simulink model "saturn_ib_stack_test"  (Simulink 6.2)
settings: Solver=ode4  SolverMode=SingleTasking  StartTime=-20.0  StopTime=620  FixedStep=0.005  RelTol=1e-3
values from neighbouring files (symbols this model uses):
  A_z_deg = 82.8200    (= 82.82)    [AS205_presettings.m]
  BN_1_sec = 14.4    [AS205_presettings.m]
  DeltaV_b_mps = 7.2381    [AS205_presettings.m]
  epsilon_2_sec = 15.0    (= 15)    [AS205_presettings.m]
  epsilon_prime_sec = 3.0    (= 3)    [AS205_presettings.m]
  i_deg = 28.89597    [AS205_presettings.m]
  lambda_0_deg = 102.32900    (= 102.329)    [AS205_presettings.m]
  lambda_L_deg = -80.561141    [AS205_presettings.m]
  pad_roll_L_deg = 100.0    (= 100)    [AS205_presettings.m]
  phi_L_deg = 28.521963    [AS205_presettings.m]
  phi_L_prime_deg = 28.360795    [AS205_presettings.m]
  R_L_m = 6373385.0    (= 6373385)    [AS205_presettings.m]
  R_T_m = 6570774.0    (= 6570774)    [AS205_presettings.m]
  T3_FM_sec = 6.08    [AS205_presettings.m]
  T_HSL_sec = 5.0    (= 5)    [AS205_presettings.m]
  Theta_T_deg = 0.000    (= 0)    [AS205_presettings.m]
  V_T_mps = 7780.976    [AS205_presettings.m]
  Xdotdot_VGT_mps2 = -9.251    [AS205_presettings.m]
undefined symbols (not defined in the file or in its folder): e0_0, e1_0, e2_0, e3_0, m, s
libraries: simulink x99, aerolibconvert x83, aerolibutil x63, aerolibtransform2 x34, aerolibasang x2, aerolibatmos2 x2, aerolib6dofsys x2
(part 2 of 7)

== system saturn_ib_stack_test/Saturn_IB_Stack/Saturn Instrument Unit (IU) ==
  note: Per Astrionics System Handbook
      | the D/A converters feeding this signal
      | into the Flight Control Computer  have
      | a quantization unit of 0.06 degrees
  note: Early Apollo technical documents use different axes assignments
      | for the Body, Gimbal, and S-Frames.
      | Documents for the AS-205 flight use the original
      | standard.  This model uses the assignments used later in the
      | project as those match up with the 1992 AIAA standard and what's
      | used in the 1972 S-IB Equation Defining Document.
  note: Control System Gain Switch Points
  ST124M_GRR_orientation_DCM : Inport  Port=1  LatchInput=off
  bS_IB_propellant_sensor_dry : Inport  Port=2  DataType=boolean  LatchInput=off
  bLiftoff : Inport  Port=3  PortDimensions=1  DataType=boolean  LatchInput=off
  phi_dot_rad_per_sec : Inport  Port=4  LatchInput=off
  A_b_mps2 : Inport  Port=5  LatchInput=off
  veh_q_ECI : Inport  Port=6  LatchInput=off
  Accelerometers : Subsystem
  Body Rate Gyros : Subsystem
  Constant3 : Constant  Value=true  OutDataTypeMode=boolean
  Constant4 : Constant  Value=true  OutDataTypeMode=boolean
  Control Error Signals : Scope  NumInputPorts=3
      settings: TimeRange=300  YMin=-1.3~-0.8~-0.07  YMax=0.7~1.1~0.05  SaveName=ScopeData6  Decimation=10  SampleTime=0.01
  Flight Control Computer : Subsystem
  Ground : Ground
  LVDA / LVDC : Subsystem
  Mux2 : Mux  Inputs=8
  ST-124M Stabilized Platform : Subsystem
  Switchpoint 1 : simulink/Logic and Bit Operations/Compare To Constant  relop=>=  const=40.0  LogicOutDataTypeMode=boolean  ZeroCross=off
  Switchpoint 2 : simulink/Logic and Bit Operations/Compare To Constant  relop=>=  const=100.0  LogicOutDataTypeMode=boolean  ZeroCross=off
  Switchpoint 3 : simulink/Logic and Bit Operations/Compare To Constant  relop=>=  const=140.0  LogicOutDataTypeMode=boolean  ZeroCross=off
  S_IB_beta_c_deg : Outport
  S_IVB_beta_c_deg : Outport  Port=2
  bS_IB_IECO : Outport  Port=3
  bS_IB_OECO : Outport  Port=4
  bS_IB_EngineStart : Outport  Port=5
  bS_IB_Stage_Sep : Outport  Port=6
  bS_IVB_UllageMotorStart : Outport  Port=7
  bS_IVB_EngineStart : Outport  Port=8
  S_IVB_APS_III_Relays : Outport  Port=9  PortDimensions=3  DataType=boolean
  S_IVB_APS_I_Relays : Outport  Port=10  PortDimensions=3  DataType=boolean
  R_S_bar_m : Outport  Port=11
  bS-IVB Cutoff : Outport  Port=12
  bSimulink_S-IVB_Enable : Outport  Port=13
  bSimulink_S-IB_Enable : Outport  Port=14
  tag scope: Psi_deg=global, S_IV_Burn=global, S_IV_Coast=global, bSwitchpoint5=global
  wires:
  Accelerometers/1(gamma_mps2) -> Control Error Signals/3, Flight Control Computer/4(gamma_mps2)
  Body Rate Gyros/1(phi_dot_deg_per_sec) -> Control Error Signals/2, Flight Control Computer/3(phi_dot_dps)
  [T1_sec] -> Flight Control Computer/1(T_sec)
  Flight Control Computer/1(s_ib_beta_c_deg) -> S_IB_beta_c_deg/1  "Beta_c"
  phi_dot_rad_per_sec/1 -> Body Rate Gyros/1(In1)
  veh_q_ECI/1 -> ST-124M Stabilized Platform/1(q_ECI)
  ST124M_GRR_orientation_DCM/1 -> ST-124M Stabilized Platform/2(ST124M DCM)
  bS_IB_propellant_sensor_dry/1 -> LVDA / LVDC/3(bSIBPropellantSensorDry)
  LVDA / LVDC/5(bIECO) -> bS_IB_IECO/1
  LVDA / LVDC/3(bSIVEngineStart) -> bS_IVB_EngineStart/1
  Flight Control Computer/3(S_IVB_APS_III_Relays) -> S_IVB_APS_III_Relays/1
  Flight Control Computer/4(S_IVB_APS_I_Relays) -> S_IVB_APS_I_Relays/1
  Constant3/1 -> bSimulink_S-IB_Enable/1
  [S_IV_Burn] -> Flight Control Computer/5(S_IV_Burn)
  [S_IV_Coast] -> Flight Control Computer/6(S_IV_Coast)
  LVDA / LVDC/8(bUllageMotorStart) -> bS_IVB_UllageMotorStart/1
  Flight Control Computer/2(s_ivb_beta_c_deg) -> S_IVB_beta_c_deg/1
  Switchpoint 1/1 -> Flight Control Computer/7(bSwitchpoint1)
  Switchpoint 2/1 -> Flight Control Computer/8(bSwitchpoint2)
  Switchpoint 3/1 -> Flight Control Computer/9(bSwitchpoint3)
  LVDA / LVDC/10(bSIVCoast) -> [S_IV_Coast]
  Ground/1 -> Flight Control Computer/10(bSwitchpoint4)
  Mux2/1 -> bS_IB_EngineStart/1
  Constant4/1 -> Mux2/1, Mux2/2, Mux2/3, Mux2/4, Mux2/5, Mux2/6, Mux2/7, Mux2/8
  A_b_mps2/1 -> Accelerometers/1(A_b_mps2), ST-124M Stabilized Platform/3(A_b_mps2)
  ST-124M Stabilized Platform/2(accumulated velocity (m/sec)) -> LVDA / LVDC/2(V_m_bar_mps)
  LVDA / LVDC/11(bSwitchpoin5) -> [bSwitchpoint5]
  [bSwitchpoint5] -> Flight Control Computer/11(bSwitchpoint5)
  LVDA / LVDC/2(Psi_deg) -> Control Error Signals/1, Flight Control Computer/2(psi_deg), [Psi_deg]
  LVDA / LVDC/4(bSIVCutoff) -> bS-IVB Cutoff/1
  LVDA / LVDC/1(R_S_bar_m) -> R_S_bar_m/1
  ST-124M Stabilized Platform/1(Gimbal Angles (deg)) -> LVDA / LVDC/1(Theta_deg)
  LVDA / LVDC/13(T1_sec) -> Switchpoint 1/1, Switchpoint 2/1, Switchpoint 3/1
  LVDA / LVDC/6(bSimulinkSIVBEnable) -> bSimulink_S-IVB_Enable/1
  LVDA / LVDC/7(bOECO) -> bS_IB_OECO/1
  LVDA / LVDC/9(bSIVBurn) -> [S_IV_Burn]
  LVDA / LVDC/12(bSIBStageSep) -> bS_IB_Stage_Sep/1
  bLiftoff/1 -> LVDA / LVDC/4(bLiftoff)

== system saturn_ib_stack_test/Saturn_IB_Stack/CM_ISS/Stable Member Gimbal Angles ==
  note: Q1 = {{Cos[IGA], 0, -Sin[IGA]}, {0, 1, 0}, {Sin[IGA], 0, Cos[IGA]}}
      | Q2 =  {{Cos[MGA],  Sin[MGA], 0}, {-Sin[MGA], Cos[MGA], 0}, {0, 0, 1}}
      | Q3 = {{1, 0, 0}, {0, Cos[OGA],  Sin[OGA]}, {0, -Sin[OGA], Cos[OGA]}}
      | Q3.Q2.Q1 = {{Cos[IGA] Cos[MGA],  Sin[MGA], -Cos[MGA] Sin[IGA]},
      |                      {-Cos[IGA] Cos[OGA] Sin[MGA] +
      |       Sin[IGA] Sin[OGA], Cos[MGA] Cos[OGA],
      |     Cos[OGA] Sin[IGA] Sin[MGA] + Cos[IGA] Sin[OGA]}, {Cos[OGA] Sin[IGA] +
      |       Cos[IGA] Sin[MGA] Sin[OGA], -Cos[MGA] Sin[OGA],
      |     Cos[IGA] Cos[OGA] - Sin[IGA] Sin[MGA] Sin[OGA]}}
  DCM : Inport  Port=1  LatchInput=off
  -Cos[MGA] Sin[OGA] : Fcn  Expr=-u(8)
  -sin(IGA)cos(MGA) : Fcn  Expr=-u(3)
  Cos[MGA] Cos[OGA] : Fcn  Expr=u(5)
  Mux2 : Mux  Inputs=3
  "Reshape 3x3 -> 9x1" : simulink/Math Operations/Reshape  OutputDimensionality=Customize  OutputDimensions=[9, 1]
  Trigonometric Function1 : Trigonometry  Operator=atan2
  Trigonometric Function3 : Trigonometry  Operator=atan2
  Trigonometric Function4 : Trigonometry  Operator=asin
  cos(IGA)cos(MGA) : Fcn  Expr=u(1)
  "sin(MGA) " : Fcn  Expr=u(2)
  CM IMU Gimbal : Outport  InitialOutput=0
  wires:
  DCM/1 -> "Reshape 3x3 -> 9x1"/1
  "Reshape 3x3 -> 9x1"/1 -> -Cos[MGA] Sin[OGA]/1, Cos[MGA] Cos[OGA]/1, -sin(IGA)cos(MGA)/1, cos(IGA)cos(MGA)/1, "sin(MGA) "/1
  -Cos[MGA] Sin[OGA]/1 -> Trigonometric Function1/1
  Cos[MGA] Cos[OGA]/1 -> Trigonometric Function1/2
  -sin(IGA)cos(MGA)/1 -> Trigonometric Function3/1
  cos(IGA)cos(MGA)/1 -> Trigonometric Function3/2
  Mux2/1 -> CM IMU Gimbal/1
  "sin(MGA) "/1 -> Trigonometric Function4/1
  Trigonometric Function4/1 -> Mux2/2  "MGA"
  Trigonometric Function3/1 -> Mux2/1  "IGA"
  Trigonometric Function1/1 -> Mux2/3  "OGA"

== system saturn_ib_stack_test/Saturn_IB_Stack/CM_ISS/Stable Member Gimbal Angles1 ==
  note: Q1 = {{Cos[IGA], 0, -Sin[IGA]}, {0, 1, 0}, {Sin[IGA], 0, Cos[IGA]}}
      | Q2 =  {{Cos[MGA],  Sin[MGA], 0}, {-Sin[MGA], Cos[MGA], 0}, {0, 0, 1}}
      | Q3 = {{1, 0, 0}, {0, Cos[OGA],  Sin[OGA]}, {0, -Sin[OGA], Cos[OGA]}}
      | Q3.Q2.Q1 = {{Cos[IGA] Cos[MGA],  Sin[MGA], -Cos[MGA] Sin[IGA]},
      |                      {-Cos[IGA] Cos[OGA] Sin[MGA] +
      |       Sin[IGA] Sin[OGA], Cos[MGA] Cos[OGA],
      |     Cos[OGA] Sin[IGA] Sin[MGA] + Cos[IGA] Sin[OGA]}, {Cos[OGA] Sin[IGA] +
      |       Cos[IGA] Sin[MGA] Sin[OGA], -Cos[MGA] Sin[OGA],
      |     Cos[IGA] Cos[OGA] - Sin[IGA] Sin[MGA] Sin[OGA]}}
  DCM : Inport  Port=1  LatchInput=off
  -Cos[MGA] Sin[OGA] : Fcn  Expr=-u(8)
  -sin(IGA)cos(MGA) : Fcn  Expr=-u(3)
  Cos[MGA] Cos[OGA] : Fcn  Expr=u(5)
  Mux2 : Mux  Inputs=3
  "Reshape 3x3 -> 9x1" : simulink/Math Operations/Reshape  OutputDimensionality=Customize  OutputDimensions=[9, 1]
  Trigonometric Function1 : Trigonometry  Operator=atan2
  Trigonometric Function3 : Trigonometry  Operator=atan2
  Trigonometric Function4 : Trigonometry  Operator=asin
  cos(IGA)cos(MGA) : Fcn  Expr=u(1)
  "sin(MGA) " : Fcn  Expr=u(2)
  CM IMU Gimbal : Outport  InitialOutput=0
  wires:
  DCM/1 -> "Reshape 3x3 -> 9x1"/1
  "Reshape 3x3 -> 9x1"/1 -> -Cos[MGA] Sin[OGA]/1, Cos[MGA] Cos[OGA]/1, -sin(IGA)cos(MGA)/1, cos(IGA)cos(MGA)/1, "sin(MGA) "/1
  -Cos[MGA] Sin[OGA]/1 -> Trigonometric Function1/1
  Cos[MGA] Cos[OGA]/1 -> Trigonometric Function1/2
  -sin(IGA)cos(MGA)/1 -> Trigonometric Function3/1
  cos(IGA)cos(MGA)/1 -> Trigonometric Function3/2
  Mux2/1 -> CM IMU Gimbal/1
  "sin(MGA) "/1 -> Trigonometric Function4/1
  Trigonometric Function4/1 -> Mux2/2  "MGA"
  Trigonometric Function3/1 -> Mux2/1  "IGA"
  Trigonometric Function1/1 -> Mux2/3  "OGA"

== system saturn_ib_stack_test/Saturn_IB_Stack/Initial Conditions/Date to JD ==
  note: Indirectly from Meeus via Vallado's "Fundamentals of Astrodynamics and Applications",
      | Second Edition
  Date  (YYYY,mm,dd,hh,mm,ss.s) : Inport  Port=1  LatchInput=off
  Add : Sum  Inputs=+++  OutScaling=2^-10
  B : Fcn  Expr=2.0 - floor(u(1)/100.0) + floor(floor( u(1)/100 )/4.0)
  Bias : Bias  Bias=-1.0
  Bias1 : Bias  Bias=12.0
  Bias2 : Bias  Bias=-1524.5
  C : Fcn  Expr=(((u(6)/60.0)+u(5))/60.0+u(4))/24.0
  C1 : Fcn  Expr=floor(365.25*(u(1)+4716)) + floor(30.6001*(u(2)+1)) + u(3)
  Compare To Constant : simulink/Logic and Bit Operations/Compare To Constant  relop=<=  const=2  LogicOutDataTypeMode=uint8  ZeroCross=off
  Demux : Demux  Outputs=6
  Mux : Mux  Inputs=6
  Switch : Switch  Criteria=u2 ~= 0
  Switch1 : Switch  Criteria=u2 ~= 0
  JD : Outport
  wires:
  Date  (YYYY,mm,dd,hh,mm,ss.s)/1 -> Demux/1
  Demux/5 -> Mux/5
  Compare To Constant/1 -> Switch1/2, Switch/2
  Bias/1 -> Switch/1
  Demux/1 -> Bias/1, Switch/3
  Bias1/1 -> Switch1/1
  Demux/2 -> Bias1/1, Switch1/3, Compare To Constant/1
  Switch/1 -> Mux/1
  Switch1/1 -> Mux/2
  Demux/3 -> Mux/3
  Demux/4 -> Mux/4
  Demux/6 -> Mux/6
  Mux/1 -> B/1, C/1, C1/1
  B/1 -> Bias2/1
  C/1 -> Add/2
  Bias2/1 -> Add/1
  Add/1 -> JD/1
  C1/1 -> Add/3

== system saturn_ib_stack_test/Saturn_IB_Stack/Initial Conditions/Initial Position and Velocity (Eqns. 3.4.3-4) ==
  R_L_m : Inport  Port=1  PortDimensions=1  LatchInput=off
  A_z_deg : Inport  Port=2  LatchInput=off
  phi_L_deg : Inport  Port=3  LatchInput=off
  phi_L_prime_deg : Inport  Port=4  LatchInput=off
  Add : Sum  Inputs=+-  OutScaling=2^-10
  Angle Conversion : aerolibconvert/Angle Conversion  IU=deg  OU=rad
  Angle Conversion1 : aerolibconvert/Angle Conversion  IU=deg  OU=rad
  Angle Conversion2 : aerolibconvert/Angle Conversion  IU=deg  OU=rad
  Fcn : Fcn  Expr=u(1)*u(7)
  Fcn1 : Fcn  Expr=u(1)*u(6)*u(2)
  Fcn2 : Fcn  Expr=-u(1)*u(6)*u(3)
  Fcn3 : Fcn  Expr=0.0
  Fcn4 : Fcn  Expr=u(1)*omega_E_rps*pi*u(9)*u(3)
  Fcn5 : Fcn  Expr=u(1)*omega_E_rps*pi*u(9)*u(2)
  Mux : Mux  Inputs=9
  Mux1 : Mux  Inputs=3
  Mux2 : Mux  Inputs=3
  SinCos{1..4} (4 alike) : aerolibutil/SinCos
  R_S_0_m : Outport
  V_S_0_mps : Outport  Port=2
  wires:
  A_z_deg/1 -> Angle Conversion/1
  Angle Conversion/1 -> SinCos1/1
  phi_L_deg/1 -> Angle Conversion1/1
  Angle Conversion1/1 -> SinCos2/1, Add/1
  R_L_m/1 -> Mux/1
  SinCos1/1 -> Mux/2
  SinCos1/2 -> Mux/3
  SinCos2/1 -> Mux/4
  SinCos2/2 -> Mux/5
  phi_L_prime_deg/1 -> Angle Conversion2/1
  Angle Conversion2/1 -> Add/2, SinCos4/1
  Add/1 -> SinCos3/1
  SinCos3/1 -> Mux/6
  SinCos3/2 -> Mux/7
  Fcn/1 -> Mux1/1
  Fcn1/1 -> Mux1/2
  Fcn2/1 -> Mux1/3
  Mux/1 -> Fcn/1, Fcn1/1, Fcn2/1, Fcn3/1, Fcn4/1, Fcn5/1
  Mux1/1 -> R_S_0_m/1
  Fcn3/1 -> Mux2/1
  Fcn4/1 -> Mux2/2
  Fcn5/1 -> Mux2/3
  Mux2/1 -> V_S_0_mps/1
  SinCos4/1 -> Mux/8
  SinCos4/2 -> Mux/9

== system saturn_ib_stack_test/Saturn_IB_Stack/Initial Conditions/L/V Inertial Orientation ==
  A_z_deg : Inport  Port=1  LatchInput=off
  phi_L_deg : Inport  Port=2  LatchInput=off
  Theta_E_deg : Inport  Port=3  LatchInput=off
  Angle Conversion2 : aerolibconvert/Angle Conversion  IU=deg  OU=rad
  E-Frame to s-Frame (MES matrix) : Subsystem  AncestorBlock="aerolibtransform2/Euler Angles to  Direction Cosine Matrix"
      mask Type: Euler2DCM
      mask Description: Determine the 3-by-3 direction cosine matrix (DCM) transforming the E-frame to the S-Frame
      mask Display: disp('MES')
  Mux : Mux  Inputs=3
  DCM : Outport
  wires:
  phi_L_deg/1 -> Mux/2
  Theta_E_deg/1 -> Mux/3
  A_z_deg/1 -> Mux/1
  Mux/1 -> Angle Conversion2/1
  E-Frame to s-Frame (MES matrix)/1(DCM) -> DCM/1
  Angle Conversion2/1 -> E-Frame to s-Frame (MES matrix)/1(Az phi_L Theta_E)

== system saturn_ib_stack_test/Saturn_IB_Stack/Initial Conditions/LLA to ECF ==
  lat (rad) : Inport  Port=1  LatchInput=off
  lon (rad) : Inport  Port=2  LatchInput=off
  h (m) : Inport  Port=3  LatchInput=off
  Add : Sum  OutScaling=2^-10
  Add1 : Sum  OutScaling=2^-10
  Bias : Bias  Bias=1.0
  Divide : Product  Inputs=*/  OutScaling=2^-10
  Divide1 : Product  Inputs=*/  OutScaling=2^-10
  Math Function : Math  Operator=square  SaturateOnIntegerOverflow=on
  Math Function1 : Math  Operator=square  SaturateOnIntegerOverflow=on
  Math Function2 : Math  Operator=square  SaturateOnIntegerOverflow=on
  Math Function3 : Math  Operator=sqrt  SaturateOnIntegerOverflow=on
  Mux : Mux  Inputs=3
  Product : Product  RndMeth=Zero
  Product1 : Product  Inputs=3  RndMeth=Zero
  Product2 : Product  Inputs=3  RndMeth=Zero
  Product3 : Product  RndMeth=Zero
  Product4 : Product  RndMeth=Zero
  SinCos : aerolibutil/SinCos
  SinCos1 : aerolibutil/SinCos
  Unary Minus : simulink/Math Operations/Unary Minus  DoSatur=off
  WGS-84 ECC^2 : Constant  Value=0.006694380004260806515  OutDataTypeMode=double
  WGS-84 major : Constant  Value=6378137.0  OutDataTypeMode=double
  WGS-84 minor : Constant  Value=6356752.3142  OutDataTypeMode=double
  XYZ (m) : Outport
  wires:
  WGS-84 major/1 -> Divide/1, Math Function2/1
  SinCos/1 -> Math Function/1, Product4/2
  WGS-84 ECC^2/1 -> Product/1
  Math Function/1 -> Product/2
  Product/1 -> Unary Minus/1
  Divide/1 -> Add/1, Product3/2  "N"
  h (m)/1 -> Add1/2, Add/2
  lat (rad)/1 -> SinCos/1
  lon (rad)/1 -> SinCos1/1
  Add/1 -> Product1/1, Product2/1
  SinCos/2 -> Product2/2, Product1/2
  SinCos1/2 -> Product1/3
  SinCos1/1 -> Product2/3
  Product1/1 -> Mux/1
  Mux/1 -> XYZ (m)/1
  Product2/1 -> Mux/2
  Product4/1 -> Mux/3
  WGS-84 minor/1 -> Math Function1/1
  Divide1/1 -> Product3/1
  Product3/1 -> Add1/1
  Add1/1 -> Product4/1
  Bias/1 -> Math Function3/1
  Unary Minus/1 -> Bias/1
  Math Function3/1 -> Divide/2
  Math Function1/1 -> Divide1/1
  Math Function2/1 -> Divide1/2

== system saturn_ib_stack_test/Saturn_IB_Stack/Initial Conditions/MES Transform ==
  theta_GMST_0_deg : Inport  Port=1  LatchInput=off
  Constant2 : Constant  Value=A_z_deg
  Constant8 : Constant  Value=phi_L_deg
  Constant9 : Constant  Value=lambda_L_deg
  MES Transform : Subsystem  TreatAsAtomicUnit=on  SystemSampleTime=0.8
  Sum2 : Sum  Inputs=|++
  DCM : Outport
  wires:
  Constant2/1 -> MES Transform/1(A_z_deg)
  Constant8/1 -> MES Transform/2(phi_L_deg)
  Constant9/1 -> Sum2/1
  Sum2/1 -> MES Transform/3(Theta_E_deg)
  theta_GMST_0_deg/1 -> Sum2/2
  MES Transform/1(DCM) -> DCM/1

== system saturn_ib_stack_test/Saturn_IB_Stack/Initial Conditions/T to GMST ==
  T_UT1 : Inport  Port=1  LatchInput=off
  Math Function : Math  Operator=mod  SaturateOnIntegerOverflow=on
  eqn : Fcn  Expr=67310.54841 + (876600*3600 + 8640184.81266) * u(1) + 0.093104*u(1)^2 - 6.2E-06 * u(1)^3
  one day : Constant  Value=86400
  seconds to degrees : Gain  Gain=1 / 240.0
  theta_GMST : Outport
  wires:
  T_UT1/1 -> eqn/1
  one day/1 -> Math Function/2
  eqn/1 -> Math Function/1
  Math Function/1 -> seconds to degrees/1
  seconds to degrees/1 -> theta_GMST/1

== system saturn_ib_stack_test/Saturn_IB_Stack/MES Transform/MES Transform ==
  A_z_deg : Inport  Port=1  LatchInput=off
  phi_L_deg : Inport  Port=2  LatchInput=off
  Theta_E_deg : Inport  Port=3  LatchInput=off
  Angle Conversion2 : aerolibconvert/Angle Conversion  IU=deg  OU=rad
  E-Frame to s-Frame (MES matrix) : Subsystem  AncestorBlock="aerolibtransform2/Euler Angles to  Direction Cosine Matrix"
      mask Type: Euler2DCM
      mask Description: Determine the 3-by-3 direction cosine matrix (DCM) transforming the E-frame to the S-Frame
      mask Display: disp('MES')
  Mux : Mux  Inputs=3
  DCM : Outport
  wires:
  phi_L_deg/1 -> Mux/2
  Theta_E_deg/1 -> Mux/3
  A_z_deg/1 -> Mux/1
  Mux/1 -> Angle Conversion2/1
  E-Frame to s-Frame (MES matrix)/1(DCM) -> DCM/1
  Angle Conversion2/1 -> E-Frame to s-Frame (MES matrix)/1(Az phi_L Theta_E)

== system saturn_ib_stack_test/Saturn_IB_Stack/On Pad/Centrifugal Acceleration ==
  Xe_m : Inport  Port=1  LatchInput=off
  ECItoBody : Inport  Port=2  LatchInput=off
  3x3 Cross Product : aerolibutil/3x3 Cross Product
  3x3 Cross Product1 : aerolibutil/3x3 Cross Product
  Product1 : Product  Multiplication=Matrix(*)  RndMeth=Zero
  omega_E_rad_per_sec : Constant  Value=[0.0 0.0 7.292115E-05]
  Out1 : Outport
  wires:
  omega_E_rad_per_sec/1 -> 3x3 Cross Product/1, 3x3 Cross Product1/1
  3x3 Cross Product/1 -> 3x3 Cross Product1/2
  3x3 Cross Product1/1 -> Product1/2
  ECItoBody/1 -> Product1/1
  Xe_m/1 -> 3x3 Cross Product/2
  Product1/1 -> Out1/1

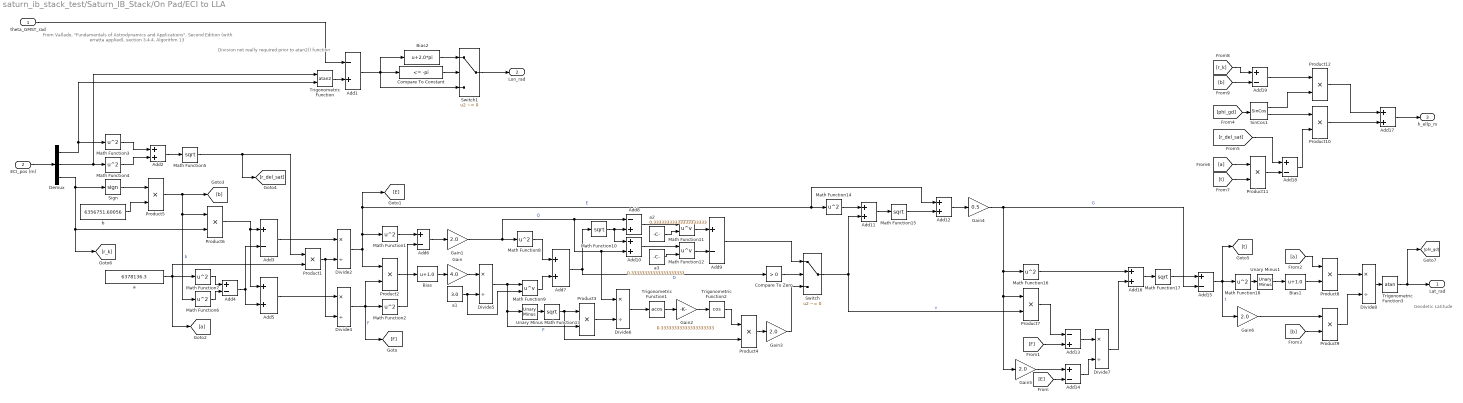
== system saturn_ib_stack_test/Saturn_IB_Stack/On Pad/ECI to LLA ==
  note: Division not really required
      | prior to atan2() function
  note: From Vallado, "Fundamentals of Astrodynamics and Applications",
      | Second Edition (with erratta applied), section 3.4.4, Algorithm 13
  note: Geodetic Latitude
  theta_GMST_rad : Inport  Port=1  LatchInput=off
  ECI_pos (m) : Inport  Port=2  LatchInput=off
  Add1 : Sum  Inputs=-+  OutScaling=2^-10
  Add{2,5,7,10..12,16..17} (8 alike) : Sum  OutScaling=2^-10
  Add13 : Sum  Inputs=-+  OutScaling=2^-10
  Add{3..4,6,9,14..15,18..19} (8 alike) : Sum  Inputs=+-  OutScaling=2^-10
  Add8 : Sum  Inputs=-+  OutScaling=2^-10
  Bias : Bias  Bias=1.0
  Bias1 : Bias  Bias=1.0
  Bias2 : Bias  Bias=2.0*pi
  Compare To Constant : simulink/Logic and Bit Operations/Compare To Constant  relop=<=  const=-pi  LogicOutDataTypeMode=boolean  ZeroCross=off
  Compare To Zero : simulink/Logic and Bit Operations/Compare To Zero  relop=>  LogicOutDataTypeMode=boolean  ZeroCross=off
  Demux : Demux  Outputs=3
  Divide{2,4..8} (6 alike) : Product  Inputs=*/  OutScaling=2^-10
  Gain : Gain  Gain=4.0
  Gain{1,3,5..6} (4 alike) : Gain  Gain=2.0
  Gain2 : Gain  Gain=0.33333333333333333333
  Gain4 : Gain  Gain=0.5
  Math Function{1..4,6..8,14,16,18} (10 alike) : Math  Operator=square  SaturateOnIntegerOverflow=on
  Math Function{5,10,13,15,17} (5 alike) : Math  Operator=sqrt  SaturateOnIntegerOverflow=on
  Math Function11 : Math  Operator=pow  SaturateOnIntegerOverflow=on
  Math Function12 : Math  Operator=pow  SaturateOnIntegerOverflow=on
  Math Function9 : Math  Operator=pow  SaturateOnIntegerOverflow=on
  Product{1..12} (12 alike) : Product  RndMeth=Zero
  Sign : Signum
  SinCos1 : aerolibutil/SinCos
  Switch : Switch  Criteria=u2 ~= 0
  Switch1 : Switch  Criteria=u2 ~= 0
  Trigonometric Function : Trigonometry  Operator=atan2
  Trigonometric Function1 : Trigonometry  Operator=acos
  Trigonometric Function2 : Trigonometry  Operator=cos
  Trigonometric Function3 : Trigonometry  Operator=atan
  Unary Minus : simulink/Math Operations/Unary Minus  DoSatur=off
  Unary Minus1 : simulink/Math Operations/Unary Minus  DoSatur=off
  a : Constant  Value=6378136.3  OutDataTypeMode=double
  a1 : Constant  Value=3.0  OutDataTypeMode=double
  a2 : Constant  Value=0.33333333333333333333  OutDataTypeMode=double
  a3 : Constant  Value=0.33333333333333333333  OutDataTypeMode=double
  b : Constant  Value=6356751.60056  OutDataTypeMode=double
  Lat_rad : Outport
  Lon_rad : Outport  Port=2
  h_ellp_m : Outport  Port=3
  wires:
  ECI_pos (m)/1 -> Demux/1
  Demux/1 -> Math Function3/1, Trigonometric Function/2
  Demux/2 -> Math Function4/1, Trigonometric Function/1
  Math Function3/1 -> Add2/1
  Math Function4/1 -> Add2/2
  Add2/1 -> Math Function5/1
  Demux/3 -> Sign/1, Product6/2, [r_k]
  Sign/1 -> Product5/1
  b/1 -> Product5/2
  Product5/1 -> Product6/1, Math Function6/1, [b]  "b"
  Product6/1 -> Add3/1, Add5/1
  Math Function6/1 -> Add4/2
  Math Function7/1 -> Add4/1
  a/1 -> Math Function7/1, Product1/2, [a]
  Add4/1 -> Add3/2, Add5/2
  Add3/1 -> Divide2/1
  Math Function5/1 -> Product1/1, [r_del_sat]
  Divide2/1 -> Product2/1, Math Function1/1, Math Function14/1, Add12/1, [E]  "E"
  Trigonometric Function/1 -> Add1/2
  theta_GMST_rad/1 -> Add1/1
  Product1/1 -> Divide2/2, Divide4/2
  Add5/1 -> Divide4/1
  Divide4/1 -> Product2/2, Math Function2/1, [F]  "F"
  Product2/1 -> Bias/1
  Bias/1 -> Gain/1
  Gain/1 -> Divide5/1
  a1/1 -> Divide5/2, Math Function9/2
  Divide5/1 -> Math Function9/1, Unary Minus/1, Product3/2  "P"
  Math Function1/1 -> Add6/1
  Math Function2/1 -> Add6/2
  Add6/1 -> Gain1/1
  Gain1/1 -> Math Function8/1, Add8/1, Add10/2, Divide6/1  "Q"
  Math Function8/1 -> Add7/1
  Math Function9/1 -> Add7/2
  Compare To Zero/1 -> Switch/2
  Add7/1 -> Compare To Zero/1, Math Function10/1  "D"
  Math Function10/1 -> Add8/2, Add10/1
  Add8/1 -> Math Function11/1
  a2/1 -> Math Function11/2
  Math Function11/1 -> Add9/1
  a3/1 -> Math Function12/2
  Math Function12/1 -> Add9/2
  Add10/1 -> Math Function12/1
  Add9/1 -> Switch/1
  Unary Minus/1 -> Math Function13/1
  Math Function13/1 -> Product3/1, Product4/2
  Product3/1 -> Divide6/2
  Divide6/1 -> Trigonometric Function1/1
  Trigonometric Function1/1 -> Gain2/1
  Gain2/1 -> Trigonometric Function2/1
  Trigonometric Function2/1 -> Product4/1
  Product4/1 -> Gain3/1
  Gain3/1 -> Switch/3
  Math Function14/1 -> Add11/1
  Switch/1 -> Add11/2, Product7/2  "v"
  Add11/1 -> Math Function15/1
  Math Function15/1 -> Add12/2
  Add12/1 -> Gain4/1
  Gain4/1 -> Math Function16/1, Product7/1, Gain5/1, Add15/2  "G"
  Product7/1 -> Add13/1
  [F] -> Add13/2
  Gain5/1 -> Add14/1
  [E] -> Add14/2
  Add13/1 -> Divide7/1
  Add14/1 -> Divide7/2
  Math Function16/1 -> Add16/1
  Divide7/1 -> Add16/2
  Add16/1 -> Math Function17/1
  Math Function17/1 -> Add15/1
  Add15/1 -> Math Function18/1, Gain6/1, [t]  "t"
  Math Function18/1 -> Unary Minus1/1
  Unary Minus1/1 -> Bias1/1
  Bias1/1 -> Product8/2
  [a] -> Product8/1
  Product8/1 -> Divide8/1
  Gain6/1 -> Product9/1
  Product9/1 -> Divide8/2
  [b] -> Product9/2
  Divide8/1 -> Trigonometric Function3/1
  Trigonometric Function3/1 -> Lat_rad/1, [phi_gd]
  [phi_gd] -> SinCos1/1
  Add17/1 -> h_ellp_m/1
  SinCos1/2 -> Product10/1
  [a] -> Product11/1
  [t] -> Product11/2
  Product11/1 -> Add18/2
  [r_del_sat] -> Add18/1
  Add18/1 -> Product10/2
  Product10/1 -> Add17/2
  [r_k] -> Add19/1
  [b] -> Add19/2
  Add19/1 -> Product12/1
  Product12/1 -> Add17/1
  SinCos1/1 -> Product12/2
  Add1/1 -> Compare To Constant/1, Bias2/1, Switch1/3
  Switch1/1 -> Lon_rad/1
  Compare To Constant/1 -> Switch1/2
  Bias2/1 -> Switch1/1

== system saturn_ib_stack_test/Saturn_IB_Stack/On Pad/Earth Gravity Model ==
  note: Gravity model accounts for Earth's oblateness.  From
      | Aircraft Control and Simulation, by Stevens and Lewis
      | who cite Brittling
  ECI_pos (m) : Inport  Port=1  PortDimensions=3  LatchInput=off
  theta_GMST_rad : Inport  Port=2  PortDimensions=1  LatchInput=off
  Add : Sum  Inputs=+++  OutScaling=2^-10
  Bias : Bias  Bias=3.0
  Bias1 : Bias  Bias=1.0
  Bias2 : Bias  Bias=1.0
  Demux : Demux  Outputs=3
  Divide : Product  Inputs=**/  OutScaling=2^-10
  Divide1 : Product  Inputs=*/  OutScaling=2^-10
  Divide2 : Product  Inputs=*/  OutScaling=2^-10
  GM : Constant  Value=3.986004418e14
  Gain : Gain  Gain=5.0
  Gain1 : Gain  Gain=1.5
  J1 : Constant  Value=3.0
  J2 : Constant  Value=0.00108263
  Math Function{,1..2,6} (4 alike) : Math  Operator=square  SaturateOnIntegerOverflow=on
  Math Function3 : Math  Operator=sqrt  SaturateOnIntegerOverflow=on
  Math Function5 : Math  Operator=pow  SaturateOnIntegerOverflow=on
  Mux : Mux  Inputs=3
  Product1 : Product  RndMeth=Zero
  Product3 : Product  Inputs=3  RndMeth=Zero
  Re : Constant  Value=6378137
  Terminator : Terminator
  Trigonometric Function : Trigonometry  Operator=asin
  Unary Minus : simulink/Math Operations/Unary Minus  DoSatur=off
  Unary Minus1 : simulink/Math Operations/Unary Minus  DoSatur=off
  g (m/s^2) : Outport  PortDimensions=3
  wires:
  ECI_pos (m)/1 -> Demux/1, Product1/2
  Demux/1 -> Math Function/1
  Demux/2 -> Math Function1/1
  Demux/3 -> Math Function2/1, Divide1/1
  Math Function/1 -> Add/1
  Math Function1/1 -> Add/2
  Math Function2/1 -> Add/3
  Add/1 -> Math Function3/1
  Divide1/1 -> Trigonometric Function/1
  Trigonometric Function/1 -> Gain/1
  Gain/1 -> Unary Minus1/1
  Unary Minus1/1 -> Bias1/1, Bias/1
  Re/1 -> Divide2/1
  Bias1/1 -> Mux/3, Mux/2
  Bias/1 -> Mux/1
  J2/1 -> Gain1/1
  Gain1/1 -> Product3/2
  Mux/1 -> Product3/3
  Divide2/1 -> Math Function6/1
  Math Function3/1 -> Divide2/2, Divide1/2, Math Function5/1
  GM/1 -> Divide/1
  Divide/1 -> Unary Minus/1
  Math Function5/1 -> Divide/3
  J1/1 -> Math Function5/2
  Unary Minus/1 -> g (m/s^2)/1
  Product3/1 -> Bias2/1
  Math Function6/1 -> Product3/1
  Bias2/1 -> Product1/1
  Product1/1 -> Divide/2
  theta_GMST_rad/1 -> Terminator/1

== system saturn_ib_stack_test/Saturn_IB_Stack/On Pad/Initial Conditions ==
  Theta_GMST_rad : Inport  Port=1  LatchInput=off
  CG_LLA_deg_m : Inport  Port=2  LatchInput=off
  3x3 Cross Product : aerolibutil/3x3 Cross Product
  Angle Conversion : aerolibconvert/Angle Conversion  IU=deg  OU=rad
  Angle Conversion1 : aerolibconvert/Angle Conversion  IU=deg  OU=rad
  Angle Conversion2 : aerolibconvert/Angle Conversion  IU=deg  OU=rad
  Angle Conversion3 : aerolibconvert/Angle Conversion  IU=rad  OU=deg
  Demux : Demux  Outputs=3
  Direction Cosine Matrix  to Quaternion : aerolibtransform2/Direction Cosine Matrix  to Quaternions
  Euler Angles to  Direction Cosine Matrix : aerolibtransform2/Euler Angles to  Direction Cosine Matrix
  L/V Inertial Orientation : Subsystem  TreatAsAtomicUnit=on  SystemSampleTime=0.8
  LLA to ECF : Subsystem
  MES Transform : Subsystem
  Mux : Mux  Inputs=3
  Position 1  Azimuth (deg) : Constant  Value=pad_roll_L_deg
  Product : Product  Multiplication=Matrix(*)  RndMeth=Zero
  Product1 : Product  Multiplication=Matrix(*)  RndMeth=Zero
  Sum : Sum  Inputs=|++
  Unary Minus : simulink/Math Operations/Unary Minus  DoSatur=off
  omega_E_rad_per_sec : Constant  Value=[0.0 0.0 7.292115E-05]
  zero : Constant  Value=0
  theta_GMST_deg : Outport
  ST124M_DCM : Outport  Port=2
  q_ECI : Outport  Port=3
  Xe_m : Outport  Port=4
  Vb_mps : Outport  Port=5
  V_ECI_mps : Outport  Port=6
  wires:
  Theta_GMST_rad/1 -> Angle Conversion3/1
  Direction Cosine Matrix  to Quaternion/1 -> q_ECI/1
  Demux/1 -> Angle Conversion/1, L/V Inertial Orientation/2(phi_L_deg)  "phi_L_deg"
  Demux/2 -> Angle Conversion1/1, Sum/2  "lambda_L_deg"
  Angle Conversion/1 -> LLA to ECF/1(lat (rad))
  Angle Conversion1/1 -> LLA to ECF/2(lon (rad))
  Demux/3 -> LLA to ECF/3(h (m))
  CG_LLA_deg_m/1 -> Demux/1
  LLA to ECF/1(XYZ (m)) -> Product/2
  Product/1 -> Xe_m/1, 3x3 Cross Product/2
  Euler Angles to  Direction Cosine Matrix/1 -> Product/1
  Mux/1 -> Euler Angles to  Direction Cosine Matrix/1
  zero/1 -> Mux/1, Mux/2
  Angle Conversion2/1 -> Mux/3
  [A] -> Unary Minus/1
  omega_E_rad_per_sec/1 -> 3x3 Cross Product/1
  Product1/1 -> Vb_mps/1
  3x3 Cross Product/1 -> Product1/2, V_ECI_mps/1  "V_ECI_0_mps"
  [A] -> Sum/1, MES Transform/1(theta_GMST_0_deg)
  Sum/1 -> L/V Inertial Orientation/3(Theta_E_deg)
  L/V Inertial Orientation/1(DCM) -> Direction Cosine Matrix  to Quaternion/1, Product1/1
  Position 1  Azimuth (deg)/1 -> L/V Inertial Orientation/1(A_z_deg)
  Unary Minus/1 -> Angle Conversion2/1
  Angle Conversion3/1 -> theta_GMST_deg/1, [A]
  MES Transform/1(DCM) -> ST124M_DCM/1

== system saturn_ib_stack_test/Saturn_IB_Stack/S-IB Stage/Aerodynamic Forces and Moments ==
  note: CP relative to Sta. 100 (positive forward)
  note: Aero forces at CP
  note: I am having a tough time finding NASA aero data for the
      | Saturn IB.  Use data from NASA-TM-X-53243 "Static Aerodynamic
      | Characteristics of the Aborted Saturn IB vehicle"
  note: C.G. relative to STA. 100
      | (positive forward)
  a_mps : Inport  Port=1  LatchInput=off
  rho : Inport  Port=2  LatchInput=off
  alpha_rad : Inport  Port=3  LatchInput=off
  beta_rad : Inport  Port=4  LatchInput=off
  V_mps : Inport  Port=5  LatchInput=off
  CG_m : Inport  Port=6  LatchInput=off
  bStageSep : Inport  Port=7  DataType=boolean  LatchInput=off
  3x3 Cross Product : aerolibutil/3x3 Cross Product
  Add : Sum  Inputs=+-|  OutScaling=2^-10
  Angle Conversion : aerolibconvert/Angle Conversion  IU=rad  OU=deg
  Angle Conversion1 : aerolibconvert/Angle Conversion  IU=rad  OU=deg
  CA_T : Lookup  InputValues=[0.0, 0.5, 0.75,1.0,1.25,1.5,6.0]  OutputValues=[1.2,0.84,0.74,0.96,1.02,0.95,0.48]
  CN(alpha) : Lookup2D  RowIndex=[0,0.2,0.4,1,2,3,4.8]  ColumnIndex=[0,2,4,6,8,10,12,14,15]  OutputValues=reshape([0.00,0.00,0.00,0.00,0,0,0,0.22,0.22,0.22,0.28,0.18,0.14,0.08,0.44,0.44,0.45,0.52,0.35,0.30,0.21,0.68,0.68,0.69,0.80,0.55,0.52,0.40,0.9,0.9,0.92,1.10,0.8,0.8,0.6,1.15,1.15,1.17,1.35,1.1,1.18,0.9,1.38,1.38,1.41,1.65,1.42,1.5,1.18,1.62,1.62,1.68,1.9,1.84,1.9,1.5,1.75,1.75,1.80,2.05,2.08,2.15,1.7],7,9)
  CN(beta) : Lookup2D  RowIndex=[0,0.2,0.4,1,2,3,4.8]  ColumnIndex=[0,2,4,6,8,10,12,14,15]  OutputValues=reshape([0.00,0.00,0.00,0.00,0,0,0,0.22,0.22,0.22,0.28,0.18,0.14,0.08,0.44,0.44,0.45,0.52,0.35,0.30,0.21,0.68,0.68,0.69,0.80,0.55,0.52,0.40,0.9,0.9,0.92,1.10,0.8,0.8,0.6,1.15,1.15,1.17,1.35,1.1,1.18,0.9,1.38,1.38,1.41,1.65,1.42,1.5,1.18,1.62,1.62,1.68,1.9,1.84,1.9,1.5,1.75,1.75,1.80,2.05,2.08,2.15,1.7],7,9)
  CP (m) : Lookup  InputValues=[0.0, 0.51, 1.2,1.54, 2.14, 6.28]  OutputValues=[17.95, 17.9109, 18.2259, 20.2936, 25.3718, 35.6068]
  Constant : Constant  Value=0.0
  Divide : Product  Inputs=*/  OutScaling=2^-10
  Dynamic Pressure : aerolibasang/Dynamic Pressure
  Mux : Mux  Inputs=3
  Mux1 : Mux  Inputs=3
  Post-separation CG : Constant  Value=[369.487*0.0254 0.0 0.0]
  Product2 : Product  Inputs=3  RndMeth=Zero
  Referece Area (m^2) : Constant  Value=34.25
  Switch : Switch  Criteria=u2 ~= 0
  Unary Minus : simulink/Math Operations/Unary Minus  DoSatur=off
  Unary Minus1 : simulink/Math Operations/Unary Minus  DoSatur=off
  Unary Minus2 : simulink/Math Operations/Unary Minus  DoSatur=off
  CP_m : Outport
  F_aero_N : Outport  Port=2
  M_aero_Nm : Outport  Port=3
  qbar : Outport  Port=4
  Mach : Outport  Port=5
  wires:
  V_mps/1 -> Divide/1, Dynamic Pressure/1
  Divide/1 -> CN(alpha)/1, CN(beta)/1, CA_T/1, Mach/1, CP (m)/1  "Mach Number"
  CN(alpha)/1 -> Unary Minus1/1
  CN(beta)/1 -> Unary Minus2/1
  CA_T/1 -> Unary Minus/1
  Mux/1 -> Product2/1
  Dynamic Pressure/1 -> Product2/2, qbar/1
  a_mps/1 -> Divide/2
  rho/1 -> Dynamic Pressure/2
  alpha_rad/1 -> Angle Conversion/1
  Product2/1 -> F_aero_N/1, 3x3 Cross Product/2
  beta_rad/1 -> Angle Conversion1/1
  Unary Minus/1 -> Mux/1
  CG_m/1 -> [CG_m]
  [CG_m] -> Add/2
  3x3 Cross Product/1 -> M_aero_Nm/1
  Add/1 -> 3x3 Cross Product/1
  CP (m)/1 -> Mux1/1
  Constant/1 -> Mux1/3, Mux1/2
  Referece Area (m^2)/1 -> Product2/3
  Unary Minus1/1 -> Mux/3
  Unary Minus2/1 -> Mux/2
  Angle Conversion/1 -> CN(alpha)/2
  Angle Conversion1/1 -> CN(beta)/2
  Post-separation CG/1 -> Switch/1
  bStageSep/1 -> Switch/2
  Mux1/1 -> Switch/3
  Switch/1 -> CP_m/1, Add/1

== system saturn_ib_stack_test/Saturn_IB_Stack/S-IB Stage/Custom Variable Mass 6DoF (Quaternion) ==
  Forces : Inport  Port=1  LatchInput=off
  Moments : Inport  Port=2  LatchInput=off
  m_dot : Inport  Port=3  LatchInput=off
  mass : Inport  Port=4  LatchInput=off
  I_dot : Inport  Port=5  LatchInput=off
  I : Inport  Port=6  LatchInput=off
  initial quaternion : Inport  Port=7  LatchInput=off
  Xe_initial_m : Inport  Port=8  PortDimensions=3  LatchInput=off
  Vb_0_mps : Inport  Port=9  LatchInput=off
  Calculate DCM & Euler Angles : Subsystem  AncestorBlock=aerolib6dofsys/DCM & Euler Angles (Quaternion)
      mask Type: DCM & Euler Angles (Quaternion)
  Calculate omega_dot : Subsystem
  "Determine Force,  Mass & Inertia" : aerolib6dofsys/Mass & Inertia (custom)
  Out9 : Terminator
  Product : Product  Inputs=*/  SaturateOnIntegerOverflow=on
  Sum : Sum  Inputs=|++  SaturateOnIntegerOverflow=on
  Transpose : Math  Orientation=up  Operator=transpose  SaturateOnIntegerOverflow=on
  Vbxw : aerolibutil/3x3 Cross Product  Orientation=left
  Velocity Conversion : aerolibconvert/Velocity Conversion  IU=m/s  OU=m/s
  Velocity Conversion1 : aerolibconvert/Velocity Conversion  IU=m/s  OU=m/s
  "p,q,r " : Integrator  InitialCondition=pm_0
  "transform to Inertial axes " : Subsystem
      mask Type: Vector Transformation
      mask Display: disp('L_EB')
  ub,vb,wb : Integrator  InitialConditionSource=external  InitialCondition=Vm_0
  xe,ye,ze : Integrator  InitialConditionSource=external  InitialCondition=xme_0
  Ve : Outport
  Xe : Outport  Port=2
  Euler : Outport  Port=3
  DCM : Outport  Port=4
  Vb : Outport  Port=5
  p,q,r : Outport  Port=6
  pdot,qdot,rdot : Outport  Port=7
  Ab : Outport  Port=8
  q : Outport  Port=9
  q0 : Outport  Port=10
  wires:
  Velocity Conversion1/1 -> Ve/1
  Velocity Conversion/1 -> Vb/1
  "Determine Force,  Mass & Inertia"/3 -> Calculate omega_dot/2("I, I_dot")
  Calculate DCM & Euler Angles/2(Euler) -> Euler/1
  Vbxw/1 -> Sum/2
  ub,vb,wb/1 -> Velocity Conversion/1, "transform to Inertial axes "/1(x y z), Vbxw/1, "Determine Force,  Mass & Inertia"/1
  Sum/1 -> ub,vb,wb/1
  xe,ye,ze/1 -> Xe/1
  "transform to Inertial axes "/1(Ve) -> Velocity Conversion1/1, xe,ye,ze/1
  "p,q,r "/1 -> p,q,r/1, Vbxw/2, Calculate omega_dot/1(p q r), Calculate DCM & Euler Angles/1(p q r)
  Moments/1 -> Calculate omega_dot/3(Moments)
  Forces/1 -> "Determine Force,  Mass & Inertia"/2
  Product/1 -> Sum/1, Ab/1
  Calculate DCM & Euler Angles/1(DCM) -> DCM/1, Transpose/1
  Transpose/1 -> "transform to Inertial axes "/2(transform coefficients)
  mass/1 -> "Determine Force,  Mass & Inertia"/3
  "Determine Force,  Mass & Inertia"/2 -> Product/2
  m_dot/1 -> "Determine Force,  Mass & Inertia"/4
  "Determine Force,  Mass & Inertia"/4 -> Out9/1
  Calculate omega_dot/1(pdot qdot rdot) -> pdot,qdot,rdot/1, "p,q,r "/1
  I/1 -> "Determine Force,  Mass & Inertia"/5
  I_dot/1 -> "Determine Force,  Mass & Inertia"/6
  "Determine Force,  Mass & Inertia"/1 -> Product/1
  Calculate DCM & Euler Angles/3(q) -> q/1
  initial quaternion/1 -> Calculate DCM & Euler Angles/2(Initial quaternion), q0/1
  Xe_initial_m/1 -> xe,ye,ze/2
  Vb_0_mps/1 -> ub,vb,wb/2

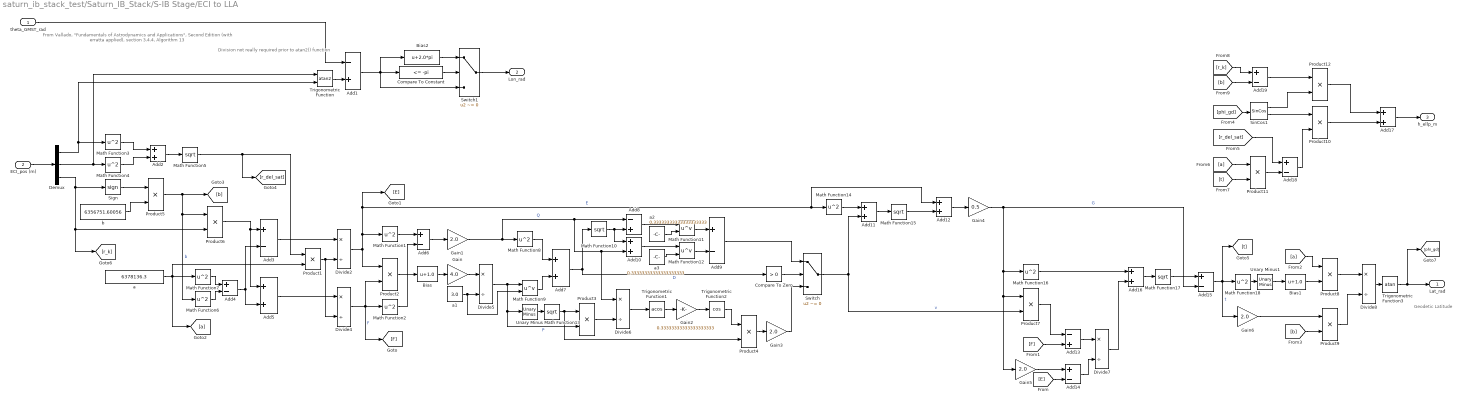
== system saturn_ib_stack_test/Saturn_IB_Stack/S-IB Stage/ECI to LLA ==
  note: Division not really required
      | prior to atan2() function
  note: From Vallado, "Fundamentals of Astrodynamics and Applications",
      | Second Edition (with erratta applied), section 3.4.4, Algorithm 13
  note: Geodetic Latitude
  theta_GMST_rad : Inport  Port=1  LatchInput=off
  ECI_pos (m) : Inport  Port=2  LatchInput=off
  Add1 : Sum  Inputs=-+  OutScaling=2^-10
  Add{2,5,7,10..12,16..17} (8 alike) : Sum  OutScaling=2^-10
  Add13 : Sum  Inputs=-+  OutScaling=2^-10
  Add{3..4,6,9,14..15,18..19} (8 alike) : Sum  Inputs=+-  OutScaling=2^-10
  Add8 : Sum  Inputs=-+  OutScaling=2^-10
  Bias : Bias  Bias=1.0
  Bias1 : Bias  Bias=1.0
  Bias2 : Bias  Bias=2.0*pi
  Compare To Constant : simulink/Logic and Bit Operations/Compare To Constant  relop=<=  const=-pi  LogicOutDataTypeMode=boolean  ZeroCross=off
  Compare To Zero : simulink/Logic and Bit Operations/Compare To Zero  relop=>  LogicOutDataTypeMode=boolean  ZeroCross=off
  Demux : Demux  Outputs=3
  Divide{2,4..8} (6 alike) : Product  Inputs=*/  OutScaling=2^-10
  Gain : Gain  Gain=4.0
  Gain{1,3,5..6} (4 alike) : Gain  Gain=2.0
  Gain2 : Gain  Gain=0.33333333333333333333
  Gain4 : Gain  Gain=0.5
  Math Function{1..4,6..8,14,16,18} (10 alike) : Math  Operator=square  SaturateOnIntegerOverflow=on
  Math Function{5,10,13,15,17} (5 alike) : Math  Operator=sqrt  SaturateOnIntegerOverflow=on
  Math Function11 : Math  Operator=pow  SaturateOnIntegerOverflow=on
  Math Function12 : Math  Operator=pow  SaturateOnIntegerOverflow=on
  Math Function9 : Math  Operator=pow  SaturateOnIntegerOverflow=on
  Product{1..12} (12 alike) : Product  RndMeth=Zero
  Sign : Signum
  SinCos1 : aerolibutil/SinCos
  Switch : Switch  Criteria=u2 ~= 0
  Switch1 : Switch  Criteria=u2 ~= 0
  Trigonometric Function : Trigonometry  Operator=atan2
  Trigonometric Function1 : Trigonometry  Operator=acos
  Trigonometric Function2 : Trigonometry  Operator=cos
  Trigonometric Function3 : Trigonometry  Operator=atan
  Unary Minus : simulink/Math Operations/Unary Minus  DoSatur=off
  Unary Minus1 : simulink/Math Operations/Unary Minus  DoSatur=off
  a : Constant  Value=6378136.3  OutDataTypeMode=double
  a1 : Constant  Value=3.0  OutDataTypeMode=double
  a2 : Constant  Value=0.33333333333333333333  OutDataTypeMode=double
  a3 : Constant  Value=0.33333333333333333333  OutDataTypeMode=double
  b : Constant  Value=6356751.60056  OutDataTypeMode=double
  Lat_rad : Outport
  Lon_rad : Outport  Port=2
  h_ellp_m : Outport  Port=3
  wires:
  ECI_pos (m)/1 -> Demux/1
  Demux/1 -> Math Function3/1, Trigonometric Function/2
  Demux/2 -> Math Function4/1, Trigonometric Function/1
  Math Function3/1 -> Add2/1
  Math Function4/1 -> Add2/2
  Add2/1 -> Math Function5/1
  Demux/3 -> Sign/1, Product6/2, [r_k]
  Sign/1 -> Product5/1
  b/1 -> Product5/2
  Product5/1 -> Product6/1, Math Function6/1, [b]  "b"
  Product6/1 -> Add3/1, Add5/1
  Math Function6/1 -> Add4/2
  Math Function7/1 -> Add4/1
  a/1 -> Math Function7/1, Product1/2, [a]
  Add4/1 -> Add3/2, Add5/2
  Add3/1 -> Divide2/1
  Math Function5/1 -> Product1/1, [r_del_sat]
  Divide2/1 -> Product2/1, Math Function1/1, Math Function14/1, Add12/1, [E]  "E"
  Trigonometric Function/1 -> Add1/2
  theta_GMST_rad/1 -> Add1/1
  Product1/1 -> Divide2/2, Divide4/2
  Add5/1 -> Divide4/1
  Divide4/1 -> Product2/2, Math Function2/1, [F]  "F"
  Product2/1 -> Bias/1
  Bias/1 -> Gain/1
  Gain/1 -> Divide5/1
  a1/1 -> Divide5/2, Math Function9/2
  Divide5/1 -> Math Function9/1, Unary Minus/1, Product3/2  "P"
  Math Function1/1 -> Add6/1
  Math Function2/1 -> Add6/2
  Add6/1 -> Gain1/1
  Gain1/1 -> Math Function8/1, Add8/1, Add10/2, Divide6/1  "Q"
  Math Function8/1 -> Add7/1
  Math Function9/1 -> Add7/2
  Compare To Zero/1 -> Switch/2
  Add7/1 -> Compare To Zero/1, Math Function10/1  "D"
  Math Function10/1 -> Add8/2, Add10/1
  Add8/1 -> Math Function11/1
  a2/1 -> Math Function11/2
  Math Function11/1 -> Add9/1
  a3/1 -> Math Function12/2
  Math Function12/1 -> Add9/2
  Add10/1 -> Math Function12/1
  Add9/1 -> Switch/1
  Unary Minus/1 -> Math Function13/1
  Math Function13/1 -> Product3/1, Product4/2
  Product3/1 -> Divide6/2
  Divide6/1 -> Trigonometric Function1/1
  Trigonometric Function1/1 -> Gain2/1
  Gain2/1 -> Trigonometric Function2/1
  Trigonometric Function2/1 -> Product4/1
  Product4/1 -> Gain3/1
  Gain3/1 -> Switch/3
  Math Function14/1 -> Add11/1
  Switch/1 -> Add11/2, Product7/2  "v"
  Add11/1 -> Math Function15/1
  Math Function15/1 -> Add12/2
  Add12/1 -> Gain4/1
  Gain4/1 -> Math Function16/1, Product7/1, Gain5/1, Add15/2  "G"
  Product7/1 -> Add13/1
  [F] -> Add13/2
  Gain5/1 -> Add14/1
  [E] -> Add14/2
  Add13/1 -> Divide7/1
  Add14/1 -> Divide7/2
  Math Function16/1 -> Add16/1
  Divide7/1 -> Add16/2
  Add16/1 -> Math Function17/1
  Math Function17/1 -> Add15/1
  Add15/1 -> Math Function18/1, Gain6/1, [t]  "t"
  Math Function18/1 -> Unary Minus1/1
  Unary Minus1/1 -> Bias1/1
  Bias1/1 -> Product8/2
  [a] -> Product8/1
  Product8/1 -> Divide8/1
  Gain6/1 -> Product9/1
  Product9/1 -> Divide8/2
  [b] -> Product9/2
  Divide8/1 -> Trigonometric Function3/1
  Trigonometric Function3/1 -> Lat_rad/1, [phi_gd]
  [phi_gd] -> SinCos1/1
  Add17/1 -> h_ellp_m/1
  SinCos1/2 -> Product10/1
  [a] -> Product11/1
  [t] -> Product11/2
  Product11/1 -> Add18/2
  [r_del_sat] -> Add18/1
  Add18/1 -> Product10/2
  Product10/1 -> Add17/2
  [r_k] -> Add19/1
  [b] -> Add19/2
  Add19/1 -> Product12/1
  Product12/1 -> Add17/1
  SinCos1/1 -> Product12/2
  Add1/1 -> Compare To Constant/1, Bias2/1, Switch1/3
  Switch1/1 -> Lon_rad/1
  Compare To Constant/1 -> Switch1/2
  Bias2/1 -> Switch1/1

== system saturn_ib_stack_test/Saturn_IB_Stack/S-IB Stage/Earth Gravity Model ==
  note: Gravity model accounts for Earth's oblateness.  From
      | Aircraft Control and Simulation, by Stevens and Lewis
      | who cite Brittling
  ECI_pos (m) : Inport  Port=1  PortDimensions=3  LatchInput=off
  theta_GMST_rad : Inport  Port=2  PortDimensions=1  LatchInput=off
  Add : Sum  Inputs=+++  OutScaling=2^-10
  Bias : Bias  Bias=3.0
  Bias1 : Bias  Bias=1.0
  Bias2 : Bias  Bias=1.0
  Demux : Demux  Outputs=3
  Divide : Product  Inputs=**/  OutScaling=2^-10
  Divide1 : Product  Inputs=*/  OutScaling=2^-10
  Divide2 : Product  Inputs=*/  OutScaling=2^-10
  GM : Constant  Value=3.986004418e14
  Gain : Gain  Gain=5.0
  Gain1 : Gain  Gain=1.5
  J1 : Constant  Value=3.0
  J2 : Constant  Value=0.00108263
  Math Function{,1..2,6} (4 alike) : Math  Operator=square  SaturateOnIntegerOverflow=on
  Math Function3 : Math  Operator=sqrt  SaturateOnIntegerOverflow=on
  Math Function5 : Math  Operator=pow  SaturateOnIntegerOverflow=on
  Mux : Mux  Inputs=3
  Product1 : Product  RndMeth=Zero
  Product3 : Product  Inputs=3  RndMeth=Zero
  Re : Constant  Value=6378137
  Terminator : Terminator
  Trigonometric Function : Trigonometry  Operator=asin
  Unary Minus : simulink/Math Operations/Unary Minus  DoSatur=off
  Unary Minus1 : simulink/Math Operations/Unary Minus  DoSatur=off
  g (m/s^2) : Outport  PortDimensions=3
  wires:
  ECI_pos (m)/1 -> Demux/1, Product1/2
  Demux/1 -> Math Function/1
  Demux/2 -> Math Function1/1
  Demux/3 -> Math Function2/1, Divide1/1
  Math Function/1 -> Add/1
  Math Function1/1 -> Add/2
  Math Function2/1 -> Add/3
  Add/1 -> Math Function3/1
  Divide1/1 -> Trigonometric Function/1
  Trigonometric Function/1 -> Gain/1
  Gain/1 -> Unary Minus1/1
  Unary Minus1/1 -> Bias1/1, Bias/1
  Re/1 -> Divide2/1
  Bias1/1 -> Mux/3, Mux/2
  Bias/1 -> Mux/1
  J2/1 -> Gain1/1
  Gain1/1 -> Product3/2
  Mux/1 -> Product3/3
  Divide2/1 -> Math Function6/1
  Math Function3/1 -> Divide2/2, Divide1/2, Math Function5/1
  GM/1 -> Divide/1
  Divide/1 -> Unary Minus/1
  Math Function5/1 -> Divide/3
  J1/1 -> Math Function5/2
  Unary Minus/1 -> g (m/s^2)/1
  Product3/1 -> Bias2/1
  Math Function6/1 -> Product3/1
  Bias2/1 -> Product1/1
  Product1/1 -> Divide/2
  theta_GMST_rad/1 -> Terminator/1

== system saturn_ib_stack_test/Saturn_IB_Stack/S-IB Stage/H-1 Engine Cluster ==
  note: Engines start commands are
      | staggered on the S-IB.
  note: Individual engine performance estimates have been integrated
      | into this model.  See NASA-CR-95967 for the orignal values.
  T0_sec : Inport  Port=1  LatchInput=off
  CG_m : Inport  Port=2  LatchInput=off
  beta_R_deg : Inport  Port=3  LatchInput=off
  beta_P_deg : Inport  Port=4  LatchInput=off
  beta_Y_deg : Inport  Port=5  LatchInput=off
  bIECO : Inport  Port=6  PortDimensions=1  DataType=boolean  LatchInput=off
  bOECO : Inport  Port=7  PortDimensions=1  DataType=boolean  LatchInput=off
  bEngineStart : Inport  Port=8  PortDimensions=8  DataType=boolean  LatchInput=off
  Add2 : Sum  Inputs=++++++++  OutScaling=2^-10
  Add3 : Sum  Inputs=++++++++  OutScaling=2^-10
  Add4 : Sum  Inputs=++++++++  OutScaling=2^-10
  Demux : Demux  Outputs=8
  Engine 1 : Subsystem  mask{mpr_deg=0, r_m=[0.0 -1.704 1.704]}
      mask prompts: mpr_deg "Mount Point Rotation (deg)"; r_m "Mount Point Location (m) [X,Y,Z] relative to Sta. 100"
  Engine 2 : Subsystem  mask{mpr_deg=-90, r_m=[0.0  -1.704 -1.704]}
      mask prompts: mpr_deg "Mount Point Rotation (deg)"; r_m "Mount Point Location (m) [X,Y,Z] relative to Sta. 100"
  Engine 3 : Subsystem  mask{mpr_deg=-180, r_m=[0.0  1.704 -1.704]}
      mask prompts: mpr_deg "Mount Point Rotation (deg)"; r_m "Mount Point Location (m) [X,Y,Z] relative to Sta. 100"
  Engine 4 : Subsystem  mask{mpr_deg=-270.0, r_m=[0.0  1.704 1.704]}
      mask prompts: mpr_deg "Mount Point Rotation (deg)"; r_m "Mount Point Location (m) [X,Y,Z] relative to Sta. 100"
  Engine 5 : Subsystem
  Engine 6 : Subsystem
  Engine 7 : Subsystem
  Engine 8 : Subsystem
  Sum10 : Sum  Inputs=|++
  Sum11 : Sum  Inputs=|-+
  Sum12 : Sum  Inputs=|++
  Sum13 : Sum  Inputs=|--
  Sum6 : Sum  Inputs=|--
  Sum7 : Sum  Inputs=|+-
  Sum8 : Sum  Inputs=|+-
  Sum9 : Sum  Inputs=|-+
  Unary Minus : simulink/Math Operations/Unary Minus  DoSatur=off
  Fb_N : Outport
  Mb_Nm : Outport  Port=2
  mdot_kg_per_sec : Outport  Port=3
  wires:
  T0_sec/1 -> Engine 2/1(T0_sec), Engine 3/1(T0_sec), Engine 4/1(T0_sec), Engine 8/1(T0_sec), Engine 7/1(T0_sec), Engine 6/1(T0_sec), Engine 5/1(T0_sec), Engine 1/1(T0_sec)
  Engine 5/2(Moment_Nm) -> Add3/5
  Engine 5/1(Thrust_N) -> Add2/5
  Engine 1/2(M_Nm) -> Add3/1
  Engine 1/1(F_N) -> Add2/1
  Engine 6/1(Thrust_N) -> Add2/6
  Engine 7/1(Thrust_N) -> Add2/7
  Engine 8/1(Thrust_N) -> Add2/8
  Engine 6/2(Moment_Nm) -> Add3/6
  Engine 7/2(Moment_Nm) -> Add3/7
  Engine 8/2(Moment_Nm) -> Add3/8
  Engine 2/1(F_N) -> Add2/2
  Engine 3/1(F_N) -> Add2/3
  Engine 4/1(F_N) -> Add2/4
  Engine 2/2(M_Nm) -> Add3/2
  Engine 4/2(M_Nm) -> Add3/4
  Engine 3/2(M_Nm) -> Add3/3
  Add4/1 -> Unary Minus/1
  Engine 8/3(mdot_kg_sec) -> Add4/8
  Engine 7/3(mdot_kg_sec) -> Add4/7
  Engine 6/3(mdot_kg_sec) -> Add4/6
  Engine 5/3(mdot_kg_sec) -> Add4/5
  Engine 4/3(mdot_kg_sec) -> Add4/4
  Engine 3/3(mdot_kg_sec) -> Add4/3
  Engine 2/3(mdot_kg_sec) -> Add4/2
  Engine 1/3(mdot_kg_sec) -> Add4/1
  beta_R_deg/1 -> Sum11/1, Sum9/1, Sum6/1, Sum7/1, Sum8/1, Sum10/1, Sum13/1, Sum12/1
  Sum6/1 -> Engine 1/4(B_actuator_cmd_deg)
  Sum7/1 -> Engine 1/3(A_actuator_cmd_deg)
  beta_P_deg/1 -> Sum13/2, Sum9/2, Sum7/2, Sum10/2
  beta_Y_deg/1 -> Sum12/2, Sum11/2, Sum8/2, Sum6/2
  Sum8/1 -> Engine 2/3(A_actuator_cmd_deg)
  Sum9/1 -> Engine 2/4(B_actuator_cmd_deg)
  Sum11/1 -> Engine 3/4(B_actuator_cmd_deg)
  Sum10/1 -> Engine 3/3(A_actuator_cmd_deg)
  Sum13/1 -> Engine 4/4(B_actuator_cmd_deg)
  Sum12/1 -> Engine 4/3(A_actuator_cmd_deg)
  Add2/1 -> Fb_N/1
  Add3/1 -> Mb_Nm/1
  Unary Minus/1 -> mdot_kg_per_sec/1
  bIECO/1 -> Engine 5/4(bEngineCutoff), Engine 6/4(bEngineCutoff), Engine 7/4(bEngineCutoff), Engine 8/4(bEngineCutoff)
  bEngineStart/1 -> Demux/1
  bOECO/1 -> Engine 4/6(bEngineCutoff), Engine 3/6(bEngineCutoff), Engine 2/6(bEngineCutoff), Engine 1/6(bEngineCutoff)
  Demux/8 -> Engine 8/3(bEngineStart)
  Demux/6 -> Engine 6/3(bEngineStart)
  Demux/5 -> Engine 5/3(bEngineStart)
  Demux/4 -> Engine 4/5(bEngineStart)
  Demux/3 -> Engine 3/5(bEngineStart)
  Demux/2 -> Engine 2/5(bEngineStart)
  Demux/1 -> Engine 1/5(bEngineStart)
  CG_m/1 -> Engine 4/2(Cg_m), Engine 8/2(Cg_m), Engine 7/2(Cg_m), Engine 6/2(Cg_m), Engine 5/2(Cg_m), Engine 3/2(Cg_m), Engine 2/2(Cg_m), Engine 1/2(Cg_m)
  Demux/7 -> Engine 7/3(bEngineStart)

== system saturn_ib_stack_test/Saturn_IB_Stack/S-IB Stage/Relative Wind ==
  Xe_m : Inport  Port=1  LatchInput=off
  B_b : Inport  Port=2  LatchInput=off
  Vb_mps : Inport  Port=3  LatchInput=off
  3x3 Cross Product : aerolibutil/3x3 Cross Product
  "Incidence, Sideslip, & Airspeed" : Subsystem  AncestorBlock=aerolibasang/Incidence, Sideslip, & Airspeed
      mask Type: Incidence,Sideslip,&Airspeed
      mask Description: Calculate the angles between the body and the velocity vector (incidence and sideslip), and the velocity magnitude from the components in body axes (Vb).
      mask Help: web(asbhelp('incidence'));
      mask Display:
      | port_label('input',1,'V_b','texmode','on');
      | port_label('output',1,'\alpha','texmode','on');
      | port_label('output',2,'\beta','texmode','on');
      | port_label('output',3,'V','texmode','on');
  Product9 : Product  Multiplication=Matrix(*)  RndMeth=Zero
  Sum6 : Sum  Inputs=-+|
  omega_E_rad_per_sec : Constant  Value=[0.0 0.0 7.292115E-05]
  alpha_rad : Outport
  beta_rad : Outport  Port=2
  V_mps : Outport  Port=3
  wires:
  omega_E_rad_per_sec/1 -> 3x3 Cross Product/1
  3x3 Cross Product/1 -> Product9/2
  Sum6/1 -> "Incidence, Sideslip, & Airspeed"/1(Vb)
  Product9/1 -> Sum6/1
  B_b/1 -> Product9/1
  "Incidence, Sideslip, & Airspeed"/1(Alpha) -> alpha_rad/1
  "Incidence, Sideslip, & Airspeed"/2(Beta) -> beta_rad/1
  Vb_mps/1 -> Sum6/2
  "Incidence, Sideslip, & Airspeed"/3(V) -> V_mps/1
  Xe_m/1 -> 3x3 Cross Product/2
